simulink model "Simultaneous_Wrist_and_Hand"  (Simulink 8.0)
settings: Solver=ode45  StartTime=0.0  StopTime=45  RelTol=1e-3
InitFcn:
  | NMF_Init;
StartFcn:
  | load('sequence.mat');
StopFcn:
  | NMF_Stop;
values from neighbouring files (symbols this model uses):
  BLremover = [0 0 0 0 0 0 0 0 0 0 0 0 ... (24 elements, 1x24)]    [BLremover.mat]    (also in Custom_NMF.m = mean(Rest_Feature_Matrix))
  H = [H_O*0.5*max(W_O);H_C*0.5*max(W_C);H_P*0.5*max(W_P);H_S*0.5*max(W_S)]    [Custom_NMF.m]    (also in H.mat = [49.1428412925 37.0160034527 32.2584684993 28.2479049409 42.)
  maxf = ones(size(Feature_Matrix,2)/8,1)    [Custom_NMF.m]    (also in maxf.mat = [1 1 1])
  NMF_threshold = -1    [NMF_threshold.mat]
  Th = [0.1 0.1 0.1 0.1]    [Custom_NMF.m]    (also in para.mat)
undefined symbols (not defined in the file or in its folder): currentCFG_Simultaneous_Wrist_and_Hand_UA, UA
undefined symbols (not defined in the file): sequence
libraries: gUSBamplib x1
settings Model: Creator=Mike  LastModifiedBy=Administrator
settings DataIOCC: SignalLoggingSaveFormat=ModelDataLogs
settings DebuggingCC: SolverPrmCheckMsg=none  FcnCallInpInsideContextMsg=UseLocalSettings
settings GRTTargetCC: CombineOutputUpdateFcns=off  GRTInterface=on

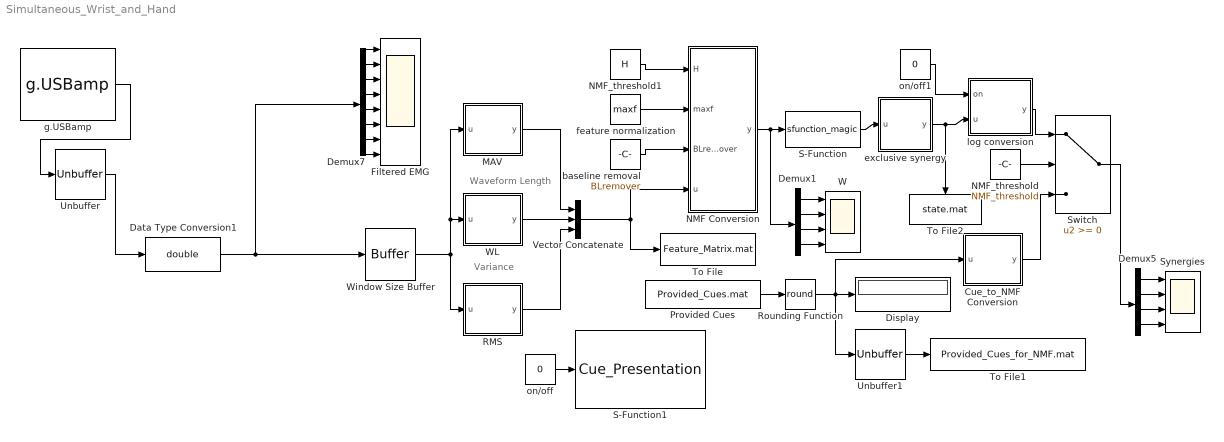
== system Simultaneous_Wrist_and_Hand ==
  note: Waveform Length
  note: Variance
  Cue_to_NMF Conversion : MATLAB Function  TreatAsAtomicUnit=on
  Data Type Conversion1 : DataTypeConversion  OutDataTypeStr=double
  Demux1 : Demux
  Demux5 : Demux
  Demux7 : Demux  Outputs=8
  Display : Display
  Filtered EMG : Scope  NumInputPorts=8
      settings: TimeRange=9  YMin=-700~-700~-700~-700~-700~-700~-700~-700  YMax=500~500~500~500~500~500~500~500  SaveName=ScopeData2
  MAV : MATLAB Function  TreatAsAtomicUnit=on
  NMF Conversion : MATLAB Function  TreatAsAtomicUnit=on
  NMF_threshold : Constant  Value=NMF_threshold  VectorParams1D=off
  NMF_threshold1 : Constant  Value=H  VectorParams1D=off
  Provided Cues : FromFile  FileName=Provided_Cues.mat  SampleTime=.001
  RMS : MATLAB Function  TreatAsAtomicUnit=on
  Rounding Function : Rounding  Operator=round  SampleTime=0.025
  S-Function : S-Function  FunctionName=sfunction_magic  Parameters=Th,NMF_threshold  EnableBusSupport=off  mask{Th=Th, NMF_threshold=NMF_threshold}
      mask prompts: Th "baseline threshold"; NMF_threshold "on/off"
  S-Function1 : S-Function  FunctionName=Cue_Presentation  Parameters=sequence  EnableBusSupport=off  mask{sequence=sequence}
      mask init:
      | Cue_Initialize;
  Switch : Switch
  Synergies : Scope  NumInputPorts=4
      settings: TimeRange=9  YMin=-0.1~-0.1~-0.1~-0.1  YMax=1.1~1.1~1.1~1.1  SaveName=ScopeData4
  To File : ToFile  Filename=Feature_Matrix.mat  MatrixName=Feature_Matrix
  To File1 : ToFile  Filename=Provided_Cues_for_NMF.mat  MatrixName=Provided_Cues
  To File2 : ToFile  Filename=state.mat  MatrixName=state
  Unbuffer : Unbuffer  SampleBasedProcessing=Same as frame based
  Unbuffer1 : Unbuffer  SampleBasedProcessing=Same as frame based
  Vector Concatenate : Concatenate  NumInputs=3  Mode=Multidimensional array  ConcatenateDimension=2
  W : Scope  NumInputPorts=4
      settings: TimeRange=9  YMin=-1~-1~-1~-1  YMax=2~2~2~2
  WL : MATLAB Function  TreatAsAtomicUnit=on
  Window Size Buffer : Buffer  N=100  V=85
  baseline removal : Constant  Value=BLremover  VectorParams1D=off
  exclusive synergy : MATLAB Function  TreatAsAtomicUnit=on
  feature normalization : Constant  Value=maxf  VectorParams1D=off
  g.USBamp : gUSBamplib/g.USBamp  cfg=currentCFG_Simultaneous_Wrist_and_Hand_UA-2007.02.03.cfg  snr=UA-2007.02.03
  log conversion : MATLAB Function  TreatAsAtomicUnit=on
  on/off : Constant  Value=0
  on/off1 : Constant  Value=0
  wires:
  Demux7/1 -> Filtered EMG/1
  Demux7/2 -> Filtered EMG/2
  Demux7/3 -> Filtered EMG/3
  Demux7/4 -> Filtered EMG/4
  Demux7/5 -> Filtered EMG/5
  Demux7/6 -> Filtered EMG/6
  Demux7/7 -> Filtered EMG/7
  Demux7/8 -> Filtered EMG/8
  MAV/1(y) -> Vector Concatenate/1
  WL/1(y) -> Vector Concatenate/2
  RMS/1(y) -> Vector Concatenate/3
  Provided Cues/1 -> Rounding Function/1
  g.USBamp/1 -> Unbuffer/1
  NMF_threshold/1 -> Switch/2
  Cue_to_NMF Conversion/1(y) -> Switch/3
  NMF_threshold1/1 -> NMF Conversion/1(H)
  Switch/1 -> Demux5/1
  on/off/1 -> S-Function1/1
  Demux5/1 -> Synergies/1
  Demux5/2 -> Synergies/2
  Demux5/3 -> Synergies/3
  Demux5/4 -> Synergies/4
  feature normalization/1 -> NMF Conversion/2(maxf)
  Vector Concatenate/1 -> NMF Conversion/4(u), To File/1
  Unbuffer1/1 -> To File1/1
  on/off1/1 -> log conversion/1(on)
  log conversion/1(y) -> Switch/1
  Rounding Function/1 -> Unbuffer1/1, Cue_to_NMF Conversion/1(u), Display/1
  baseline removal/1 -> NMF Conversion/3(BLremover)
  Window Size Buffer/1 -> MAV/1(u), WL/1(u), RMS/1(u)
  Unbuffer/1 -> Data Type Conversion1/1
  Data Type Conversion1/1 -> Demux7/1, Window Size Buffer/1
  Demux1/1 -> W/1
  Demux1/2 -> W/2
  Demux1/3 -> W/3
  Demux1/4 -> W/4
  exclusive synergy/1(y) -> To File2/1, log conversion/2(u)
  NMF Conversion/1(y) -> S-Function/1, Demux1/1
  S-Function/1 -> exclusive synergy/1(u)

== matlab function MAV ==
  data: u input double; y output double
function y = fcn(u)
%#codegen

y = mean(abs(u));

== matlab function NMF Conversion ==
  data: H input double; maxf input double; BLremover input double; u input double; y output double
function y = fcn(H,maxf,BLremover,u)
%#codegen

% normalization
u=u-BLremover;
j=1;
for i=1:8:length(u)
    u(i:i+7)=u(i:i+7)/maxf(j);
    j=j+1;
end

y = u/H;

== matlab function WL ==
  data: u input double; y output double
function y = fcn(u)
%#codegen

% y = zeros(1,size(u,2));
% for j=1:1:size(u,2)
%     temp_WL = 0;
%     for i=1:1:size(u,1)-1
%         temp_WL = temp_WL + abs(u(i+1,j)-u(i,j));
%     end
%     y(j) = temp_WL;
% end

y = sum(abs(diff(u)));

== matlab function RMS ==
  data: u input double; y output double
function y = fcn(u)
%#codegen

y = sqrt(var(u));

== matlab function Cue_to_NMF Conversion ==
  data: u input double; y output double
function y = fcn(u)
%#codegen

switch u
    case 1 % Rest
        y=[0 0 0 0];
    case 2 % Open
        y=[1 0 0 0];
    case 3 % Close
        y=[0 1 0 0];
    case 8 % Open Pronate
        y=[1 0 1 0];
    case 9 % Close Pronate
        y=[0 1 1 0];
    case 6 % Open Supinate
        y=[1 0 0 1];
    case 7 % Close Supinate
        y=[0 1 0 1];
    case 4 % Pronate
        y=[0 0 1 0];
    case 5 % Supinate
        y=[0 0 0 1];
    otherwise
        y=[0 0 0 0];
end

== matlab function log conversion ==
  data: on input double; u input double; y output double
function y = takelog(on,u)
%#codegen

if on==1
    y = log10(u*9+1);
else
    y=u;
end

== matlab function exclusive synergy ==
  data: u input double; y output double
function y = fcn(u)
%#codegen

y=u;
% if mode == 1
    if y(1)>y(2)
        y(2)=0;
    else 
        y(1)=0;
    end
    if y(3)>y(4)
        y(4)=0;
    else 
        y(3)=0;
    end
% elseif mode == 2
%     if y(1)>y(2)
%         y(1)=y(1)-y(2);
%         y(2)=0;
%     else
%         y(2)=y(2)-y(1);
%         y(1)=0;
%     end
%     if y(3)>y(4)
%         y(3)=y(3)-y(4);
%         y(4)=0;
%     else
%         y(4)=y(4)-y(3);
%         y(3)=0;
%     end
% end
